simulink model "ES101A_DiagcMgr"  (R2013b)
settings: Solver=ode45  StartTime=0.0  StopTime=0.44  RelTol=1e-3
values from neighbouring files (symbols this model uses):
  BrdgVltg = DataDict.IpSignal    [ES101A_DiagcMgr_DataDict.m]
  DEM_CLEAR_PENDING = DataDict.Constant    [ES101A_DiagcMgr_DataDict.m]
  DEM_DTC_GROUP_ALL_DTCS = DataDict.Constant    [ES101A_DiagcMgr_DataDict.m]
  DFTAGICNTR_CNT_U08 = DataDict.Constant    [ES101A_DiagcMgr_DataDict.m]
  DIAGCMGR_NTCINFOSTSTESTFAILD_CNT_U08 = DataDict.Constant    [ES101A_DiagcMgrProxyX_DataDict.m]    (also in ES101A_DiagcMgr_DataDict.m)
  DIAGCMGR_NTCINFOSTSTESTFAILDTHISIGNCYC_CNT_U08 = DataDict.Constant    [ES101A_DiagcMgr_DataDict.m]
  DIAGCMGR_NTCINFOSTSTESTNOTCMPLTHISIGNCYC_CNT_U08 = DataDict.Constant    [ES101A_DiagcMgrProxyX_DataDict.m]    (also in ES101A_DiagcMgr_DataDict.m)
  DiagcMgrFltResp = DataDict.Calibration    [ES101A_DiagcMgrProxyX_DataDict.m]    (also in ES101A_DiagcMgr_DataDict.m)
  DiagcMgrNtcFltAry = DataDict.NVM    [ES101A_DiagcMgr_DataDict.m]
  DIAGCSTSCTRLDSHTDWNFLTPRSNT_CNT_U16 = DataDict.Constant    [ES101A_DiagcMgr_DataDict.m]
  DIAGCSTSDFTHWAG_CNT_U16 = DataDict.Constant    [ES101A_DiagcMgr_DataDict.m]
  DIAGCSTSDFTHWAGSERLCOMEXPRTVAL_CNT_U16 = DataDict.Constant    [ES101A_DiagcMgr_DataDict.m]
  DIAGCSTSDFTVEHSPD_CNT_U16 = DataDict.Constant    [ES101A_DiagcMgr_DataDict.m]
  DIAGCSTSININVAL_CNT_U16 = DataDict.Constant    [ES101A_DiagcMgrProxyX_DataDict.m]    (also in ES101A_DiagcMgr_DataDict.m)
  DIAGCSTSIVTR1INACTV_CNT_U16 = DataDict.Constant    [ES101A_DiagcMgr_DataDict.m]
  DIAGCSTSIVTR2INACTV_CNT_U16 = DataDict.Constant    [ES101A_DiagcMgr_DataDict.m]
  DIAGCSTSLIMDTPRFMNC_CNT_U16 = DataDict.Constant    [ES101A_DiagcMgr_DataDict.m]
  DIAGCSTSRAMPTOZEROFLTPRSNT_CNT_U16 = DataDict.Constant    [ES101A_DiagcMgr_DataDict.m]
  DIAGCSTSWHLIMBREJCTNDI_CNT_U16 = DataDict.Constant    [ES101A_DiagcMgr_DataDict.m]
  DTCIDXSTSFAIL_CNT_U08 = DataDict.Constant    [ES101A_DiagcMgr_DataDict.m]
  DTCIDXSTSNONTC_CNT_U08 = DataDict.Constant    [ES101A_DiagcMgr_DataDict.m]
  DTCIDXSTSNORES_CNT_U08 = DataDict.Constant    [ES101A_DiagcMgr_DataDict.m]
  DTCIDXSTSPASS_CNT_U08 = DataDict.Constant    [ES101A_DiagcMgr_DataDict.m]
  DTCIDXSTSUPDCFMD_CNT_U08 = DataDict.Constant    [ES101A_DiagcMgr_DataDict.m]
  ELECGLBPRM_IVTRCNT_CNT_U08 = DataDict.ConfigParam    [ES101A_DiagcMgrProxyX_DataDict.m]    (also in ES101A_DiagcMgr_DataDict.m)
  FLTINJ_DIAGCMGR_DIAGCSTSIVTR1INACTV = DataDict.Constant    [ES101A_DiagcMgr_DataDict.m]
  FLTINJ_DIAGCMGR_DIAGCSTSIVTR2INACTV = DataDict.Constant    [ES101A_DiagcMgr_DataDict.m]
  HwTq = DataDict.IpSignal    [ES101A_DiagcMgr_DataDict.m]
  IgnCntr = DataDict.IpSignal    [ES101A_DiagcMgr_DataDict.m]
  MAXDEBCNTRVAL_CNT_S16 = DataDict.Constant    [ES101A_DiagcMgr_DataDict.m]
  MAXRAMPRATE_ULSPERSEC_F32 = DataDict.Constant    [ES101A_DiagcMgrProxyX_DataDict.m]    (also in ES101A_DiagcMgr_DataDict.m)
  MINDEBCNTRVAL_CNT_S16 = DataDict.Constant    [ES101A_DiagcMgr_DataDict.m]
  MINRAMPRATE_ULSPERSEC_F32 = DataDict.Constant    [ES101A_DiagcMgrProxyX_DataDict.m]    (also in ES101A_DiagcMgr_DataDict.m)
  SCAMOTTQCMDTOONE_ULS_F32 = DataDict.Constant    [ES101A_DiagcMgrProxyX_DataDict.m]    (also in ES101A_DiagcMgr_DataDict.m)
  SCAMOTTQCMDTOZERO_ULS_F32 = DataDict.Constant    [ES101A_DiagcMgrProxyX_DataDict.m]    (also in ES101A_DiagcMgr_DataDict.m)
  SysSt = DataDict.IpSignal    [ES101A_DiagcMgr_DataDict.m]
  VehSpd = DataDict.IpSignal    [ES101A_DiagcMgr_DataDict.m]
undefined symbols (not defined in the file or in its folder): ActvMotTqCmdSca, ActvRampRate, AgiCntr, Dem_DTCFormatType, Dem_DTCOriginType, Dem_EventStatusType, DiagcData, DiagcMgrNtcMap, DiagcSts, DtcEnaMask, EcuT, HistNtcFltAry, MicroDiagcData, MotTq, NtcNr, NtcNrWithResd1, NtcStInfo, ProxySetNtcData, Sts, SysSt1, TOTNROFDTC_CNT_U08
libraries: simulink x149, FloatToFixd x5, NxtrNvM x3
(part 4 of 13)

== system ES101A_DiagcMgr/DiagcMgr/ReadNtcFltAry/Update DiagcMgrReadFltInfoAry and HistReadFltAry ==
  IC : Inport
  Add : Sum
  Bus Selector1 : BusSelector  OutputSignals=ApplIdx,NtcInfoIdx
  Compare To Constant : simulink/Logic and Bit Operations/Compare To Constant  relop=<  const=20  OutDataTypeStr=boolean
  Compare To Constant1 : simulink/Logic and Bit Operations/Compare To Constant  relop=<=  const=511  OutDataTypeStr=boolean
  Constant : Constant  OutDataTypeStr=uint8
  CopyRight2 : Subsystem  Description=|  mask(Copyright Information){none=on}
      | Copyright info block.                                               
      |                                                                     
      | Place copyright information at the top of every subsystem in design.
      mask prompts: none "No parameters"
      mask help: Place copyright information at the top of every subsystem in design.
      mask Display:
      | NxtrConf = 'Nexteer Confidential';
      | 
      | sys = bdroot; %handle for the current model ("system")
      | first = get_param(sys,'Created');
      | first = first(end-3:end);  %year is last four digits
      | 
      | last = get_param(sys,'LastModifiedDate');
      | if isempty(last)
      |     last = datestr(now,'yyyy');
      | else
      |     last = last(end-3:end);
      | end
      | 
      | if strcmp(first,last)
      |     fprintf('%s -- Copyright %s Nexteer',NxtrConf,first)
      | else
      |     fprintf('%s -- %s%s- %s Nexteer',NxtrConf,char(169),first,last)
      | end
  Data Store Read1 : DataStoreRead  DataStoreName=NtcMapIdx  DataStoreElements=NtcMapIdx
  Data Store Read2 : DataStoreRead  DataStoreName=DiagcMgrNtcMap  DataStoreElements=DiagcMgrNtcMap(:)
  Data Store Read3 : DataStoreRead  DataStoreName=ReadFltInfoIdx
  Data Store Read4 : DataStoreRead  DataStoreName=NtcMapIdx
  Data Store Write1 : DataStoreWrite  DataStoreName=NtcMapIdx
  For Number of NTCs : Subsystem  TreatAsAtomicUnit=on
  Logical Operator : Logic  AllPortsSameDT=off  OutDataTypeStr=boolean
  Selector1 : Selector  IndexMode=Zero-based  InputPortWidth=512  IndexOptions=Index vector (port)  Indices=[1 3]  OutputSizes=1
  While Iterator : WhileIterator  MaxIters=511  ShowIterationPort=on
  wires:
  Data Store Read2/1 -> Selector1/1
  Selector1/1 -> Bus Selector1/1
  While Iterator/1 -> For Number of NTCs/3(NtcMapIdx), Selector1/2
  Bus Selector1/1 -> For Number of NTCs/1(ApplIdx)  "<ApplIdx>"
  IC/1 -> While Iterator/2
  Logical Operator/1 -> While Iterator/1
  Add/1 -> Data Store Write1/1
  Constant/1 -> Add/2
  Data Store Read1/1 -> Add/1
  Data Store Read3/1 -> Compare To Constant/1
  Compare To Constant/1 -> Logical Operator/1
  Compare To Constant1/1 -> Logical Operator/2
  Data Store Read4/1 -> Compare To Constant1/1
  Bus Selector1/2 -> For Number of NTCs/2(NtcInfoIdx)  "<NtcInfoIdx>"

== system ES101A_DiagcMgr/DiagcMgr/ReadNtcFltAry/While((HistReadFltAryTempIdx < HistReadFltAryIdx) AND (ReadFltInfoIndx < 20)) ==
  IC : Inport
  Add1 : Sum  Inputs=+-
  Compare To Constant3 : simulink/Logic and Bit Operations/Compare To Constant  relop=<  const=0  OutDataTypeStr=boolean
  Compare To Constant5 : simulink/Logic and Bit Operations/Compare To Constant  relop=<=  const=20  OutDataTypeStr=boolean
  CopyRight1 : Subsystem  Description=|  mask(Copyright Information){none=on}
      | Copyright info block.                                               
      |                                                                     
      | Place copyright information at the top of every subsystem in design.
      mask prompts: none "No parameters"
      mask help: Place copyright information at the top of every subsystem in design.
      mask Display:
      | NxtrConf = 'Nexteer Confidential';
      | 
      | sys = bdroot; %handle for the current model ("system")
      | first = get_param(sys,'Created');
      | first = first(end-3:end);  %year is last four digits
      | 
      | last = get_param(sys,'LastModifiedDate');
      | if isempty(last)
      |     last = datestr(now,'yyyy');
      | else
      |     last = last(end-3:end);
      | end
      | 
      | if strcmp(first,last)
      |     fprintf('%s -- Copyright %s Nexteer',NxtrConf,first)
      | else
      |     fprintf('%s -- %s%s- %s Nexteer',NxtrConf,char(169),first,last)
      | end
  Data Store Read5 : DataStoreRead  DataStoreName=HistReadFltAryIdx
  Data Store Read7 : DataStoreRead  DataStoreName=ReadFltInfoIdx
  Data Store Read8 : DataStoreRead  DataStoreName=HistReadFltAryTempIdx
  Increment HistFltAryTempdx and NtcFltAryIdx : Subsystem  Priority=2
      settings: AttributesFormatString=Priority = %<Priority>
  Logical Operator1 : Logic  AllPortsSameDT=off  OutDataTypeStr=boolean
  Update NtcFltAry : Subsystem  Priority=1
      settings: AttributesFormatString=|
      | Priority = %<Priority>
      | %<Description>
  While Iterator : WhileIterator  MaxIters=20
  wires:
  IC/1 -> While Iterator/2
  Data Store Read8/1 -> Add1/1
  Data Store Read5/1 -> Add1/2
  Add1/1 -> Compare To Constant3/1
  Data Store Read7/1 -> Compare To Constant5/1
  Compare To Constant5/1 -> Logical Operator1/1
  Compare To Constant3/1 -> Logical Operator1/2
  Logical Operator1/1 -> While Iterator/1

== system ES101A_DiagcMgr/DiagcMgr/ReadNtcFltAry/While(ReadFltInfoIdx < TableSize[DiagcMgrReadFltInfoAry]) ==
  IC : Inport
  Compare To Constant2 : simulink/Logic and Bit Operations/Compare To Constant  relop=<  const=20  OutDataTypeStr=boolean
  CopyRight1 : Subsystem  Description=|  mask(Copyright Information){none=on}
      | Copyright info block.                                               
      |                                                                     
      | Place copyright information at the top of every subsystem in design.
      mask prompts: none "No parameters"
      mask help: Place copyright information at the top of every subsystem in design.
      mask Display:
      | NxtrConf = 'Nexteer Confidential';
      | 
      | sys = bdroot; %handle for the current model ("system")
      | first = get_param(sys,'Created');
      | first = first(end-3:end);  %year is last four digits
      | 
      | last = get_param(sys,'LastModifiedDate');
      | if isempty(last)
      |     last = datestr(now,'yyyy');
      | else
      |     last = last(end-3:end);
      | end
      | 
      | if strcmp(first,last)
      |     fprintf('%s -- Copyright %s Nexteer',NxtrConf,first)
      | else
      |     fprintf('%s -- %s%s- %s Nexteer',NxtrConf,char(169),first,last)
      | end
  Data Store Read6 : DataStoreRead  DataStoreName=ReadFltInfoIdx
  Increment Indices : Subsystem  Priority=2
      settings: AttributesFormatString=%<Priority>
  Update NtcFltAry : Subsystem  Priority=1
      settings: AttributesFormatString=%<Priority>
  While Iterator : WhileIterator  MaxIters=20
  wires:
  IC/1 -> While Iterator/2
  Data Store Read6/1 -> Compare To Constant2/1
  Compare To Constant2/1 -> While Iterator/1

== system ES101A_DiagcMgr/DiagcMgr/ReadNtcInfoAndDebCntr/ApplX ==
  note: This server runnable is designed such that any NTC of the type Non-Debounced
      | that is passed as an argument to this function will get a 0 value as its DebCntr.
      | DiagcMgr inherently does not store a unique DebCntr for Non-Debounced NTCs.
      | Hence the logic.
  NtcInfoIdx_ArgIn : Inport
  DebCntrIdx_ArgIn : Inport  Port=2
  Action Port : ActionPort  ActionType=case
  CopyRight2 : Subsystem  Description=|  mask(Copyright Information){none=on}
      | Copyright info block.                                               
      |                                                                     
      | Place copyright information at the top of every subsystem in design.
      mask prompts: none "No parameters"
      mask help: Place copyright information at the top of every subsystem in design.
      mask Display:
      | NxtrConf = 'Nexteer Confidential';
      | 
      | sys = bdroot; %handle for the current model ("system")
      | first = get_param(sys,'Created');
      | first = first(end-3:end);  %year is last four digits
      | 
      | last = get_param(sys,'LastModifiedDate');
      | if isempty(last)
      |     last = datestr(now,'yyyy');
      | else
      |     last = last(end-3:end);
      | end
      | 
      | if strcmp(first,last)
      |     fprintf('%s -- Copyright %s Nexteer',NxtrConf,first)
      | else
      |     fprintf('%s -- %s%s- %s Nexteer',NxtrConf,char(169),first,last)
      | end
  Debounced : Subsystem  TreatAsAtomicUnit=on
  GetNtcInfoAppIX : Subsystem  TreatAsAtomicUnit=on
  If1 : If  IfExpression=u1 == 0
  Merge : Merge
  NonDebounced : Subsystem  TreatAsAtomicUnit=on
  NtcInfo_ArgOut : Outport
  DebCntr_ArgOut : Outport  Port=2
  wires:
  NtcInfoIdx_ArgIn/1 -> GetNtcInfoAppIX/1(NtcInfoIdx_ArgIn)
  GetNtcInfoAppIX/1(NtcInfo_ArgOut) -> NtcInfo_ArgOut/1
  DebCntrIdx_ArgIn/1 -> If1/1, Debounced/1(DebCntrIdx_ArgIn)
  If1/1 -> NonDebounced/Action
  If1/2 -> Debounced/Action
  Merge/1 -> DebCntr_ArgOut/1
  NonDebounced/1(DebCntr_ArgOut) -> Merge/1
  Debounced/1(DebCntr_ArgOut) -> Merge/2

== system ES101A_DiagcMgr/DiagcMgr/ReadNtcInfoAndDebCntr/CopyRight2 ==

== system ES101A_DiagcMgr/DiagcMgr/ReadNtcInfoAndDebCntr/DoNothing ==
  Action Port : ActionPort
  CopyRight2 : Subsystem  Description=|  mask(Copyright Information){none=on}
      | Copyright info block.                                               
      |                                                                     
      | Place copyright information at the top of every subsystem in design.
      mask prompts: none "No parameters"
      mask help: Place copyright information at the top of every subsystem in design.
      mask Display:
      | NxtrConf = 'Nexteer Confidential';
      | 
      | sys = bdroot; %handle for the current model ("system")
      | first = get_param(sys,'Created');
      | first = first(end-3:end);  %year is last four digits
      | 
      | last = get_param(sys,'LastModifiedDate');
      | if isempty(last)
      |     last = datestr(now,'yyyy');
      | else
      |     last = last(end-3:end);
      | end
      | 
      | if strcmp(first,last)
      |     fprintf('%s -- Copyright %s Nexteer',NxtrConf,first)
      | else
      |     fprintf('%s -- %s%s- %s Nexteer',NxtrConf,char(169),first,last)
      | end

== system ES101A_DiagcMgr/DiagcMgr/ReadSnpshtData/CopyRight1 ==

== system ES101A_DiagcMgr/DiagcMgr/ReadSnpshtData/Send out data ==
  CopyRight2 : Subsystem  Description=|  mask(Copyright Information){none=on}
      | Copyright info block.                                               
      |                                                                     
      | Place copyright information at the top of every subsystem in design.
      mask prompts: none "No parameters"
      mask help: Place copyright information at the top of every subsystem in design.
      mask Display:
      | NxtrConf = 'Nexteer Confidential';
      | 
      | sys = bdroot; %handle for the current model ("system")
      | first = get_param(sys,'Created');
      | first = first(end-3:end);  %year is last four digits
      | 
      | last = get_param(sys,'LastModifiedDate');
      | if isempty(last)
      |     last = datestr(now,'yyyy');
      | else
      |     last = last(end-3:end);
      | end
      | 
      | if strcmp(first,last)
      |     fprintf('%s -- Copyright %s Nexteer',NxtrConf,first)
      | else
      |     fprintf('%s -- %s%s- %s Nexteer',NxtrConf,char(169),first,last)
      | end
  Data Store Read1 : DataStoreRead  DataStoreName=SnpshtDataAry
  ReadSnpshtAry_ArgOut : Outport
  wires:
  Data Store Read1/1 -> ReadSnpshtAry_ArgOut/1

== system ES101A_DiagcMgr/DiagcMgr/RestoreNtcFltAryDft/CopyRight2 ==

== system ES101A_DiagcMgr/DiagcMgr/RestoreNtcFltAryDft/Subsystem ==
  Length of NtcFltArray : Inport
  Assignment1 : Assignment  IndexMode=Zero-based  IndexOptions=Index vector (port)  Indices=1  OutputSizes=1
  Bus Assignment1 : BusAssignment  AssignedSignals=NtcNr,AgiCntr,Sts
  Constant1 : Constant  Value=0  OutDataTypeStr=uint16
  Constant2 : Constant  Value=DFTAGICNTR_CNT_U08  OutDataTypeStr=uint8
  Constant3 : Constant  Value=0  OutDataTypeStr=uint8
  CopyRight2 : Subsystem  Description=|  mask(Copyright Information){none=on}
      | Copyright info block.                                               
      |                                                                     
      | Place copyright information at the top of every subsystem in design.
      mask prompts: none "No parameters"
      mask help: Place copyright information at the top of every subsystem in design.
      mask Display:
      | NxtrConf = 'Nexteer Confidential';
      | 
      | sys = bdroot; %handle for the current model ("system")
      | first = get_param(sys,'Created');
      | first = first(end-3:end);  %year is last four digits
      | 
      | last = get_param(sys,'LastModifiedDate');
      | if isempty(last)
      |     last = datestr(now,'yyyy');
      | else
      |     last = last(end-3:end);
      | end
      | 
      | if strcmp(first,last)
      |     fprintf('%s -- Copyright %s Nexteer',NxtrConf,first)
      | else
      |     fprintf('%s -- %s%s- %s Nexteer',NxtrConf,char(169),first,last)
      | end
  Data Store Read1 : DataStoreRead  DataStoreName=DiagcMgrNtcFltAry  DataStoreElements=DiagcMgrNtcFltAry(:)
  Data Store Write2 : DataStoreWrite  DataStoreName=DiagcMgrNtcFltAry  DataStoreElements=DiagcMgrNtcFltAry(:)
  For Iterator : ForIterator  IterationSource=external  IndexMode=Zero-based
  Selector1 : Selector  IndexMode=Zero-based  InputPortWidth=20  IndexOptions=Index vector (port)  Indices=[1 3]  OutputSizes=1
  wires:
  Constant3/1 -> Bus Assignment1/4
  Constant2/1 -> Bus Assignment1/3
  Constant1/1 -> Bus Assignment1/2
  Length of NtcFltArray/1 -> For Iterator/1
  For Iterator/1 -> Selector1/2, Assignment1/3
  Bus Assignment1/1 -> Assignment1/2
  Assignment1/1 -> Data Store Write2/1
  Selector1/1 -> Bus Assignment1/1
  Data Store Read1/1 -> Selector1/1, Assignment1/1

== system ES101A_DiagcMgr/DiagcMgr/RestoreSnpshtAryDft/CopyRight2 ==

== system ES101A_DiagcMgr/DiagcMgr/RestoreSnpshtAryDft/Subsystem ==
  Length of Snapshot Array : Inport
  Assignment1 : Assignment  IndexMode=Zero-based  IndexOptions=Index vector (port)  Indices=1  OutputSizes=1
  Bus Assignment3 : BusAssignment  AssignedSignals=MicroDiagcData,HwTq,MotTq,IgnCntr,BrdgVltg,EcuT,NtcNr,NtcStInfo,SysSt,VehSpd
  Constant1 : Constant  Value=0  OutDataTypeStr=uint32
  Constant12 : Constant  Value=0  OutDataTypeStr=uint8
  Constant{2..4,7..8} (5 alike) : Constant  Value=0  OutDataTypeStr=single
  Constant5 : Constant  Value=SysSt1.SYSST_WRMININ  OutDataTypeStr=Enum: SysSt1
  Constant6 : Constant  Value=0  OutDataTypeStr=uint32
  Constant9 : Constant  Value=NtcNrWithResd1.NTCNR_RESD  OutDataTypeStr=Enum: NtcNrWithResd1
  CopyRight2 : Subsystem  Description=|  mask(Copyright Information){none=on}
      | Copyright info block.                                               
      |                                                                     
      | Place copyright information at the top of every subsystem in design.
      mask prompts: none "No parameters"
      mask help: Place copyright information at the top of every subsystem in design.
      mask Display:
      | NxtrConf = 'Nexteer Confidential';
      | 
      | sys = bdroot; %handle for the current model ("system")
      | first = get_param(sys,'Created');
      | first = first(end-3:end);  %year is last four digits
      | 
      | last = get_param(sys,'LastModifiedDate');
      | if isempty(last)
      |     last = datestr(now,'yyyy');
      | else
      |     last = last(end-3:end);
      | end
      | 
      | if strcmp(first,last)
      |     fprintf('%s -- Copyright %s Nexteer',NxtrConf,first)
      | else
      |     fprintf('%s -- %s%s- %s Nexteer',NxtrConf,char(169),first,last)
      | end
  Data Store Read1 : DataStoreRead  DataStoreName=SnpshtDataAry
  Data Store Write2 : DataStoreWrite  DataStoreName=SnpshtDataAry
  For Iterator : ForIterator  IterationSource=external  IndexMode=Zero-based  IterationVariableDataType=int16
  Selector1 : Selector  IndexMode=Zero-based  InputPortWidth=20  IndexOptions=Index vector (port)  Indices=[1 3]  OutputSizes=1
  wires:
  Data Store Read1/1 -> Assignment1/1, Selector1/1
  Selector1/1 -> Bus Assignment3/1
  Assignment1/1 -> Data Store Write2/1
  Bus Assignment3/1 -> Assignment1/2
  For Iterator/1 -> Assignment1/3, Selector1/2
  Length of Snapshot Array/1 -> For Iterator/1
  Constant1/1 -> Bus Assignment3/2
  Constant2/1 -> Bus Assignment3/3
  Constant9/1 -> Bus Assignment3/8
  Constant5/1 -> Bus Assignment3/10
  Constant12/1 -> Bus Assignment3/9
  Constant6/1 -> Bus Assignment3/5
  Constant7/1 -> Bus Assignment3/6
  Constant8/1 -> Bus Assignment3/7
  Constant3/1 -> Bus Assignment3/4
  Constant4/1 -> Bus Assignment3/11

== system ES101A_DiagcMgr/DiagcMgr/SetNtcStsCore/CopyRight2 ==

== system ES101A_DiagcMgr/DiagcMgr/SetNtcStsCore/Create SnapshotDataBus ==
  SysSt : Inport
  IgnCntr : Inport  Port=2
  RegInBRAMDAT1 : Inport  Port=3
  HwTq : Inport  Port=4
  MotTqCmdMrfScad : Inport  Port=5
  BrdgVltg : Inport  Port=6
  EcuTFild : Inport  Port=7
  VehSpd : Inport  Port=8
  Bus Creator : BusCreator  Inputs=8  OutDataTypeStr=Bus: SnpshtDataRec1
  CopyRight2 : Subsystem  Description=|  mask(Copyright Information){none=on}
      | Copyright info block.                                               
      |                                                                     
      | Place copyright information at the top of every subsystem in design.
      mask prompts: none "No parameters"
      mask help: Place copyright information at the top of every subsystem in design.
      mask Display:
      | NxtrConf = 'Nexteer Confidential';
      | 
      | sys = bdroot; %handle for the current model ("system")
      | first = get_param(sys,'Created');
      | first = first(end-3:end);  %year is last four digits
      | 
      | last = get_param(sys,'LastModifiedDate');
      | if isempty(last)
      |     last = datestr(now,'yyyy');
      | else
      |     last = last(end-3:end);
      | end
      | 
      | if strcmp(first,last)
      |     fprintf('%s -- Copyright %s Nexteer',NxtrConf,first)
      | else
      |     fprintf('%s -- %s%s- %s Nexteer',NxtrConf,char(169),first,last)
      | end
  FloatToFixd_s16_f1 : FloatToFixd/FloatToFixd_s16_f32  Param1=10
  FloatToFixd_s16_f3 : FloatToFixd/FloatToFixd_s16_f32  Param1=7
  FloatToFixd_s16_f32 : FloatToFixd/FloatToFixd_s16_f32  Param1=10
  FloatToFixd_u16_f1 : FloatToFixd/FloatToFixd_u16_f32  Param1=7
  FloatToFixd_u16_f32 : FloatToFixd/FloatToFixd_u16_f32  Param1=10
  SnapshotDataBus : Outport
  wires:
  SysSt/1 -> Bus Creator/7
  IgnCntr/1 -> Bus Creator/1
  RegInBRAMDAT1/1 -> Bus Creator/2
  HwTq/1 -> FloatToFixd_s16_f32/1
  MotTqCmdMrfScad/1 -> FloatToFixd_s16_f1/1
  BrdgVltg/1 -> FloatToFixd_u16_f32/1
  EcuTFild/1 -> FloatToFixd_s16_f3/1
  VehSpd/1 -> FloatToFixd_u16_f1/1
  Bus Creator/1 -> SnapshotDataBus/1
  FloatToFixd_s16_f32/1 -> Bus Creator/3
  FloatToFixd_s16_f1/1 -> Bus Creator/4
  FloatToFixd_u16_f32/1 -> Bus Creator/5
  FloatToFixd_s16_f3/1 -> Bus Creator/6
  FloatToFixd_u16_f1/1 -> Bus Creator/8

== system ES101A_DiagcMgr/DiagcMgr/SetNtcStsCore/NtcNr is Invalid ==
  Action Port : ActionPort  ActionType=else
  CopyRight2 : Subsystem  Description=|  mask(Copyright Information){none=on}
      | Copyright info block.                                               
      |                                                                     
      | Place copyright information at the top of every subsystem in design.
      mask prompts: none "No parameters"
      mask help: Place copyright information at the top of every subsystem in design.
      mask Display:
      | NxtrConf = 'Nexteer Confidential';
      | 
      | sys = bdroot; %handle for the current model ("system")
      | first = get_param(sys,'Created');
      | first = first(end-3:end);  %year is last four digits
      | 
      | last = get_param(sys,'LastModifiedDate');
      | if isempty(last)
      |     last = datestr(now,'yyyy');
      | else
      |     last = last(end-3:end);
      | end
      | 
      | if strcmp(first,last)
      |     fprintf('%s -- Copyright %s Nexteer',NxtrConf,first)
      | else
      |     fprintf('%s -- %s%s- %s Nexteer',NxtrConf,char(169),first,last)
      | end
  E_NOT_OK : Constant  OutDataTypeStr=uint8
  SetNtcSts_StdRtn : Outport
  wires:
  E_NOT_OK/1 -> SetNtcSts_StdRtn/1

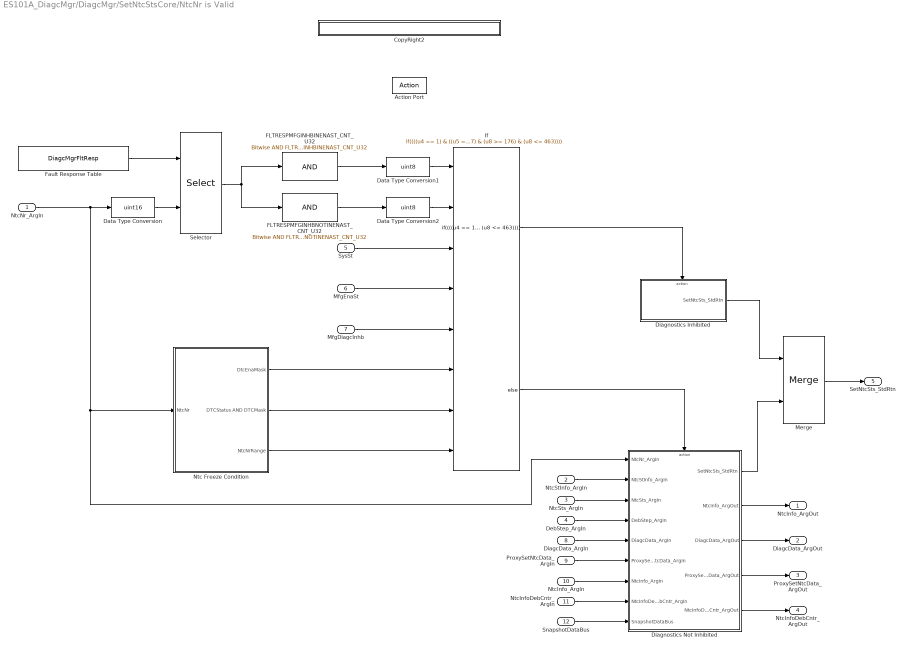
== system ES101A_DiagcMgr/DiagcMgr/SetNtcStsCore/NtcNr is Valid ==
  NtcNr_ArgIn : Inport  OutDataTypeStr=Enum: NtcNr1
  NtcStInfo_ArgIn : Inport  Port=2
  NtcSts_ArgIn : Inport  Port=3
  DebStep_ArgIn : Inport  Port=4
  SysSt : Inport  Port=5
  MfgEnaSt : Inport  Port=6
  MfgDiagcInhb : Inport  Port=7
  DiagcData_ArgIn : Inport  Port=8
  ProxySetNtcData_ArgIn : Inport  Port=9
  NtcInfo_ArgIn : Inport  Port=10
  NtcInfoDebCntr_ArgIn : Inport  Port=11
  SnapshotDataBus : Inport  Port=12
  Action Port : ActionPort  ActionType=then
  CopyRight2 : Subsystem  Description=|  mask(Copyright Information){none=on}
      | Copyright info block.                                               
      |                                                                     
      | Place copyright information at the top of every subsystem in design.
      mask prompts: none "No parameters"
      mask help: Place copyright information at the top of every subsystem in design.
      mask Display:
      | NxtrConf = 'Nexteer Confidential';
      | 
      | sys = bdroot; %handle for the current model ("system")
      | first = get_param(sys,'Created');
      | first = first(end-3:end);  %year is last four digits
      | 
      | last = get_param(sys,'LastModifiedDate');
      | if isempty(last)
      |     last = datestr(now,'yyyy');
      | else
      |     last = last(end-3:end);
      | end
      | 
      | if strcmp(first,last)
      |     fprintf('%s -- Copyright %s Nexteer',NxtrConf,first)
      | else
      |     fprintf('%s -- %s%s- %s Nexteer',NxtrConf,char(169),first,last)
      | end
  Data Type Conversion : DataTypeConversion  OutDataTypeStr=uint16
  Data Type Conversion1 : DataTypeConversion  OutDataTypeStr=uint8
  Data Type Conversion2 : DataTypeConversion  OutDataTypeStr=uint8
  Diagnostics Inhibited : Subsystem
  Diagnostics Not Inhibited : Subsystem  RequirementInfo="{'linktype_rmi_doors' '0000c474 (/ESG Group/FDD Module Requirements/EA4 Specific/ES101A_DiagcMgr)' '#ES101A_68' 'true' 'REQ:  ES101A_68' '' ; 'linktype_rmi_doors' '0000c474 (/ESG Group/FDD Module Requirements/EA4 Specific/ES101A_DiagcMgr)' '#ES101A_278' 'true' 'REQ:  ES101A_278' '' } %GIDa_b7a1320e_7113_43ee_9c12_2e59701a8c27"
  FLTRESPMFGINHBINENAST_CNT_U32 : simulink/Logic and Bit Operations/Bitwise Operator  RequirementInfo={} %GIDa_e3e71e30_edd6_46d9_83c6_38d60561c01e  logicop=AND  UseBitMask=on  BitMask=FLTRESPMFGINHBINENAST_CNT_U32  BitMaskRealWorld=Stored Integer
  FLTRESPMFGINHBNOTINENAST_CNT_U32 : simulink/Logic and Bit Operations/Bitwise Operator  RequirementInfo={} %GIDa_f5890cc9_815a_470c_bd58_76004367c247  logicop=AND  UseBitMask=on  BitMask=FLTRESPMFGINHBNOTINENAST_CNT_U32  BitMaskRealWorld=Stored Integer
  Fault Response Table : Constant  Value=DiagcMgrFltResp
  If : If  NumInputs=8  IfExpression=(((u4 == 1) & ((u5 == 1) & (u1 == 1)) | ((u2 == 1) & (u3 ~= 2))) | ((u6 ~= u7) & (u8 >= 176) & (u8 <= 463)))
  Merge : Merge
  Ntc Freeze Condition : Subsystem  RequirementInfo="{'linktype_rmi_doors' '0000c474 (/ESG Group/FDD Module Requirements/EA4 Specific/ES101A_DiagcMgr)' '#ES101A_306' 'true' 'REQ:  ES101A_306' '' ; 'linktype_rmi_doors' '0000c474 (/ESG Group/FDD Module Requirements/EA4 Specific/ES101A_DiagcMgr)' '#ES101A_316' 'true' 'REQ:  ES101A_316' '' } %GIDa_4961b6b2_f681_49a6_be60_c18be2f59728"
  Selector : Selector  IndexMode=Zero-based  InputPortWidth=512  IndexOptions=Index vector (port)  Indices=[1 3]  OutputSizes=1
  NtcInfo_ArgOut : Outport
  DiagcData_ArgOut : Outport  Port=2
  ProxySetNtcData_ArgOut : Outport  Port=3
  NtcInfoDebCntr_ArgOut : Outport  Port=4
  SetNtcSts_StdRtn : Outport  Port=5
  wires:
  NtcStInfo_ArgIn/1 -> Diagnostics Not Inhibited/2(NtcStInfo_ArgIn)
  NtcSts_ArgIn/1 -> Diagnostics Not Inhibited/3(NtcSts_ArgIn)
  DebStep_ArgIn/1 -> Diagnostics Not Inhibited/4(DebStep_ArgIn)
  Fault Response Table/1 -> Selector/1
  Selector/1 -> FLTRESPMFGINHBNOTINENAST_CNT_U32/1, FLTRESPMFGINHBINENAST_CNT_U32/1
  FLTRESPMFGINHBNOTINENAST_CNT_U32/1 -> Data Type Conversion2/1
  MfgEnaSt/1 -> If/4
  MfgDiagcInhb/1 -> If/5
  SysSt/1 -> If/3
  If/1 -> Diagnostics Inhibited/Action
  If/2 -> Diagnostics Not Inhibited/Action
  Data Type Conversion/1 -> Selector/2
  FLTRESPMFGINHBINENAST_CNT_U32/1 -> Data Type Conversion1/1
  Data Type Conversion1/1 -> If/1
  Data Type Conversion2/1 -> If/2
  DiagcData_ArgIn/1 -> Diagnostics Not Inhibited/5(DiagcData_ArgIn)
  ProxySetNtcData_ArgIn/1 -> Diagnostics Not Inhibited/6(ProxySetNtcData_ArgIn)
  NtcInfo_ArgIn/1 -> Diagnostics Not Inhibited/7(NtcInfo_ArgIn)
  Diagnostics Not Inhibited/2("NtcInfo_ArgOut ") -> NtcInfo_ArgOut/1
  Diagnostics Not Inhibited/3("DiagcData_ArgOut ") -> DiagcData_ArgOut/1
  Diagnostics Not Inhibited/4("ProxySetNtcData_ArgOut ") -> ProxySetNtcData_ArgOut/1
  NtcInfoDebCntr_ArgIn/1 -> Diagnostics Not Inhibited/8(NtcInfoDebCntr_ArgIn)
  Diagnostics Not Inhibited/5("NtcInfoDebCntr_ArgOut ") -> NtcInfoDebCntr_ArgOut/1
  Diagnostics Not Inhibited/1(SetNtcSts_StdRtn) -> Merge/2
  Diagnostics Inhibited/1(SetNtcSts_StdRtn) -> Merge/1
  Merge/1 -> SetNtcSts_StdRtn/1
  NtcNr_ArgIn/1 -> Diagnostics Not Inhibited/1(NtcNr_ArgIn), Ntc Freeze Condition/1(NtcNr), Data Type Conversion/1
  Ntc Freeze Condition/1(DtcEnaMask) -> If/6
  Ntc Freeze Condition/2(DTCStatus AND DTCMask) -> If/7
  Ntc Freeze Condition/3(NtcNrRange) -> If/8
  SnapshotDataBus/1 -> Diagnostics Not Inhibited/9(SnapshotDataBus)

== system ES101A_DiagcMgr/DiagcMgr/UpdDtcEnaCdn/ClrBit ==
  DtcEnaCdnId_ArgIn : Inport
  Action Port : ActionPort  ActionType=else
  Bitwise Operator : simulink/Logic and Bit Operations/Bitwise Operator  logicop=AND  UseBitMask=off  NumInputPorts=2  BitMask=bin2dec('11011001')  BitMaskRealWorld=Stored Integer
  Bitwise Operator1 : simulink/Logic and Bit Operations/Bitwise Operator  logicop=NOT  UseBitMask=off  BitMask=bin2dec('11011001')  BitMaskRealWorld=Stored Integer
  Constant : Constant  OutDataTypeStr=uint16
  CopyRight2 : Subsystem  Description=|  mask(Copyright Information){none=on}
      | Copyright info block.                                               
      |                                                                     
      | Place copyright information at the top of every subsystem in design.
      mask prompts: none "No parameters"
      mask help: Place copyright information at the top of every subsystem in design.
      mask Display:
      | NxtrConf = 'Nexteer Confidential';
      | 
      | sys = bdroot; %handle for the current model ("system")
      | first = get_param(sys,'Created');
      | first = first(end-3:end);  %year is last four digits
      | 
      | last = get_param(sys,'LastModifiedDate');
      | if isempty(last)
      |     last = datestr(now,'yyyy');
      | else
      |     last = last(end-3:end);
      | end
      | 
      | if strcmp(first,last)
      |     fprintf('%s -- Copyright %s Nexteer',NxtrConf,first)
      | else
      |     fprintf('%s -- %s%s- %s Nexteer',NxtrConf,char(169),first,last)
      | end
  Data Store Read : DataStoreRead  DataStoreName=DtcEnaSts
  Data Store Write : DataStoreWrite  DataStoreName=DtcEnaSts
  Shift Arithmetic : ArithShift  BitShiftNumberSource=Input port  BitShiftNumber=8  BitShiftDirection=Left
      settings: InputPortMap=u0,p1
  wires:
  DtcEnaCdnId_ArgIn/1 -> Shift Arithmetic/2
  Constant/1 -> Shift Arithmetic/1
  Bitwise Operator/1 -> Data Store Write/1
  Data Store Read/1 -> Bitwise Operator/1
  Shift Arithmetic/1 -> Bitwise Operator1/1
  Bitwise Operator1/1 -> Bitwise Operator/2

== system ES101A_DiagcMgr/DiagcMgr/UpdDtcEnaCdn/CopyRight2 ==

== system ES101A_DiagcMgr/DiagcMgr/UpdDtcEnaCdn/SetBit ==
  DtcEnaCdnId_ArgIn : Inport
  Action Port : ActionPort  ActionType=then
  Bitwise Operator : simulink/Logic and Bit Operations/Bitwise Operator  logicop=OR  UseBitMask=off  NumInputPorts=2  BitMask=bin2dec('11011001')  BitMaskRealWorld=Stored Integer
  Constant : Constant  OutDataTypeStr=uint16
  CopyRight2 : Subsystem  Description=|  mask(Copyright Information){none=on}
      | Copyright info block.                                               
      |                                                                     
      | Place copyright information at the top of every subsystem in design.
      mask prompts: none "No parameters"
      mask help: Place copyright information at the top of every subsystem in design.
      mask Display:
      | NxtrConf = 'Nexteer Confidential';
      | 
      | sys = bdroot; %handle for the current model ("system")
      | first = get_param(sys,'Created');
      | first = first(end-3:end);  %year is last four digits
      | 
      | last = get_param(sys,'LastModifiedDate');
      | if isempty(last)
      |     last = datestr(now,'yyyy');
      | else
      |     last = last(end-3:end);
      | end
      | 
      | if strcmp(first,last)
      |     fprintf('%s -- Copyright %s Nexteer',NxtrConf,first)
      | else
      |     fprintf('%s -- %s%s- %s Nexteer',NxtrConf,char(169),first,last)
      | end
  Data Store Read : DataStoreRead  DataStoreName=DtcEnaSts
  Data Store Write : DataStoreWrite  DataStoreName=DtcEnaSts
  Shift Arithmetic : ArithShift  BitShiftNumberSource=Input port  BitShiftNumber=8  BitShiftDirection=Left
      settings: InputPortMap=u0,p1
  wires:
  DtcEnaCdnId_ArgIn/1 -> Shift Arithmetic/2
  Constant/1 -> Shift Arithmetic/1
  Bitwise Operator/1 -> Data Store Write/1
  Data Store Read/1 -> Bitwise Operator/1
  Shift Arithmetic/1 -> Bitwise Operator/2

== system ES101A_DiagcMgr/DiagcMgr/ClrSnpshtData/Subsystem/CopyRight2 ==

== system ES101A_DiagcMgr/DiagcMgr/DiagcMgrIninCore/Initialize the NtcInfo Array/CopyRight2 ==

== system ES101A_DiagcMgr/DiagcMgr/DiagcMgrIninCore/Initialize the NtcInfo Array/Update the ISO bits of each NTC ==
  Number of Iteration : Inport
  NtcInfoAry_ArgIn : Inport  Port=2
  CopyRight2 : Subsystem  Description=|  mask(Copyright Information){none=on}
      | Copyright info block.                                               
      |                                                                     
      | Place copyright information at the top of every subsystem in design.
      mask prompts: none "No parameters"
      mask help: Place copyright information at the top of every subsystem in design.
      mask Display:
      | NxtrConf = 'Nexteer Confidential';
      | 
      | sys = bdroot; %handle for the current model ("system")
      | first = get_param(sys,'Created');
      | first = first(end-3:end);  %year is last four digits
      | 
      | last = get_param(sys,'LastModifiedDate');
      | if isempty(last)
      |     last = datestr(now,'yyyy');
      | else
      |     last = last(end-3:end);
      | end
      | 
      | if strcmp(first,last)
      |     fprintf('%s -- Copyright %s Nexteer',NxtrConf,first)
      | else
      |     fprintf('%s -- %s%s- %s Nexteer',NxtrConf,char(169),first,last)
      | end
  For Iterator : ForIterator  IterationSource=external  IterationLimit=22  IndexMode=Zero-based  IterationVariableDataType=int8
  Start Initialization : Subsystem  RequirementInfo="{'linktype_rmi_doors' '0000c474 (/ESG Group/FDD Module Requirements/EA4 Specific/ES101A_DiagcMgr)' '#ES101A_132' 'true' 'REQ:  ES101A_132' '' ; 'linktype_rmi_doors' '0000c474 (/ESG Group/FDD Module Requirements/EA4 Specific/ES101A_DiagcMgr)' '#ES101A_180' 'true' 'REQ:  ES101A_180' '' ; 'linktype_rmi_doors' '0000c474 (/ESG Group/FDD Module Requirements/EA4 Specific/ES101A_DiagcMgr)' '#ES101A_244' 'true' 'REQ:  ES101A_244' '' ; 'linktype_rmi_doors' '0000c474 (/ESG Group/FDD Module Requirements/EA4 Specific/ES101A_DiagcMgr)' '#ES101A_250' 'true' 'REQ:  ES101A_250' '' ; 'linktype_rmi_doors' '0000c474 (/ESG Group/FDD Module Requirements/EA4 Specific/ES101A_DiagcMgr)' '#ES101A_181' 'true' 'REQ:  ES101A_181' '' ; 'linktype_rmi_doors' '0000c474 (/ESG Group/FDD Module Requirements/EA4 Specific/ES101A_DiagcMgr)' '#ES101A_184' 'true' 'REQ:  ES101A_184' '' ; 'linktype_rmi_doors' '0000c474 (/ESG Group/FDD Module Requirements/EA4 Specific/ES101A_DiagcMgr)' '#ES101A_303' 'true' 'REQ:  ES101A_303' '' ; 'linktype_rmi_doors' '0000c474 (/ESG Group/FDD Module Requirements/EA4 Specific/ES101A_DiagcMgr)' '#ES101A_134' 'true' 'REQ:  ES101A_134' '' ; 'linktype_rmi_doors' '0000c474 (/ESG Group/FDD Module Requirements/EA4 Specific/ES101A_DiagcMgr)' '#ES101A_198' 'true' 'REQ:  ES101A_198' '' } %GIDa_7307835e_1e72_4461_aea7_7f9719f5946a"  TreatAsAtomicUnit=on
  NtcInfoAry_ArgOut : Outport
  wires:
  Number of Iteration/1 -> For Iterator/1
  For Iterator/1 -> Start Initialization/1(NtcInfoIdx)
  Start Initialization/1(NtcInfoAry_ArgOut) -> NtcInfoAry_ArgOut/1
  NtcInfoAry_ArgIn/1 -> Start Initialization/2(NtcInfoAry_ArgIn)

== system ES101A_DiagcMgr/DiagcMgr/DiagcMgrIninCore/Update DiagcSts and DiagcMgrActv/CopyRight2 ==

== system ES101A_DiagcMgr/DiagcMgr/DiagcMgrIninCore/Update DiagcSts and DiagcMgrActv/Dual Inverter ==
  Action Port : ActionPort  ActionType=else
  CopyRight2 : Subsystem  Description=|  mask(Copyright Information){none=on}
      | Copyright info block.                                               
      |                                                                     
      | Place copyright information at the top of every subsystem in design.
      mask prompts: none "No parameters"
      mask help: Place copyright information at the top of every subsystem in design.
      mask Display:
      | NxtrConf = 'Nexteer Confidential';
      | 
      | sys = bdroot; %handle for the current model ("system")
      | first = get_param(sys,'Created');
      | first = first(end-3:end);  %year is last four digits
      | 
      | last = get_param(sys,'LastModifiedDate');
      | if isempty(last)
      |     last = datestr(now,'yyyy');
      | else
      |     last = last(end-3:end);
      | end
      | 
      | if strcmp(first,last)
      |     fprintf('%s -- Copyright %s Nexteer',NxtrConf,first)
      | else
      |     fprintf('%s -- %s%s- %s Nexteer',NxtrConf,char(169),first,last)
      | end
  Inverter 2 Inactive : Constant  Value=DIAGCSTSININVAL_CNT_U16  OutDataTypeStr=uint16
  DiagcSts : Outport
  wires:
  Inverter 2 Inactive/1 -> DiagcSts/1

== system ES101A_DiagcMgr/DiagcMgr/DiagcMgrIninCore/Update DiagcSts and DiagcMgrActv/Single Inverter ==
  Action Port : ActionPort  ActionType=then
  CopyRight2 : Subsystem  Description=|  mask(Copyright Information){none=on}
      | Copyright info block.                                               
      |                                                                     
      | Place copyright information at the top of every subsystem in design.
      mask prompts: none "No parameters"
      mask help: Place copyright information at the top of every subsystem in design.
      mask Display:
      | NxtrConf = 'Nexteer Confidential';
      | 
      | sys = bdroot; %handle for the current model ("system")
      | first = get_param(sys,'Created');
      | first = first(end-3:end);  %year is last four digits
      | 
      | last = get_param(sys,'LastModifiedDate');
      | if isempty(last)
      |     last = datestr(now,'yyyy');
      | else
      |     last = last(end-3:end);
      | end
      | 
      | if strcmp(first,last)
      |     fprintf('%s -- Copyright %s Nexteer',NxtrConf,first)
      | else
      |     fprintf('%s -- %s%s- %s Nexteer',NxtrConf,char(169),first,last)
      | end
  Inverter 2 Inactive : Constant  Value=DIAGCSTSIVTR2INACTV_CNT_U16  OutDataTypeStr=uint16
  DiagcSts : Outport
  wires:
  Inverter 2 Inactive/1 -> DiagcSts/1

== system ES101A_DiagcMgr/DiagcMgr/DiagcMgrIninCore/Update NtcInfoAry From NvM/CopyRight2 ==

== system ES101A_DiagcMgr/DiagcMgr/DiagcMgrIninCore/Update NtcInfoAry From NvM/Update NtcInfoAry ==
  Length of NtcFltArray : Inport
  AppIdx_ArgIn : Inport  Port=2
  NtcInfoAry_ArgIn : Inport  Port=3
  CopyRight2 : Subsystem  Description=|  mask(Copyright Information){none=on}
      | Copyright info block.                                               
      |                                                                     
      | Place copyright information at the top of every subsystem in design.
      mask prompts: none "No parameters"
      mask help: Place copyright information at the top of every subsystem in design.
      mask Display:
      | NxtrConf = 'Nexteer Confidential';
      | 
      | sys = bdroot; %handle for the current model ("system")
      | first = get_param(sys,'Created');
      | first = first(end-3:end);  %year is last four digits
      | 
      | last = get_param(sys,'LastModifiedDate');
      | if isempty(last)
      |     last = datestr(now,'yyyy');
      | else
      |     last = last(end-3:end);
      | end
      | 
      | if strcmp(first,last)
      |     fprintf('%s -- Copyright %s Nexteer',NxtrConf,first)
      | else
      |     fprintf('%s -- %s%s- %s Nexteer',NxtrConf,char(169),first,last)
      | end
  For Iterator : ForIterator  IterationSource=external  IterationLimit=511  IndexMode=Zero-based  IterationVariableDataType=int8
  Update NtcInfoAry Aging Counter And Confirmed Bit : Subsystem  RequirementInfo={} %GIDa_5386584a_0950_4e1a_98bb_690191ebced3  TreatAsAtomicUnit=on
  NtcInfoAry_ArgOut : Outport
  wires:
  For Iterator/1 -> Update NtcInfoAry Aging Counter And Confirmed Bit/1(NtcFltIdx)
  Length of NtcFltArray/1 -> For Iterator/1
  AppIdx_ArgIn/1 -> Update NtcInfoAry Aging Counter And Confirmed Bit/2(AppIdx_ArgIn)
  NtcInfoAry_ArgIn/1 -> Update NtcInfoAry Aging Counter And Confirmed Bit/3(NtcInfoAry_ArgIn)
  Update NtcInfoAry Aging Counter And Confirmed Bit/1(NtcInfoAry_ArgOut) -> NtcInfoAry_ArgOut/1

== system ES101A_DiagcMgr/DiagcMgr/DiagcMgrPer1/Update OutpDiagcData/CopyRight2 ==

== system ES101A_DiagcMgr/DiagcMgr/DiagcMgrPer1/Update OutpDiagcData/GetDiagcDataApplX ==
  CopyRight2 : Subsystem  Description=|  mask(Copyright Information){none=on}
      | Copyright info block.                                               
      |                                                                     
      | Place copyright information at the top of every subsystem in design.
      mask prompts: none "No parameters"
      mask help: Place copyright information at the top of every subsystem in design.
      mask Display:
      | NxtrConf = 'Nexteer Confidential';
      | 
      | sys = bdroot; %handle for the current model ("system")
      | first = get_param(sys,'Created');
      | first = first(end-3:end);  %year is last four digits
      | 
      | last = get_param(sys,'LastModifiedDate');
      | if isempty(last)
      |     last = datestr(now,'yyyy');
      | else
      |     last = last(end-3:end);
      | end
      | 
      | if strcmp(first,last)
      |     fprintf('%s -- Copyright %s Nexteer',NxtrConf,first)
      | else
      |     fprintf('%s -- %s%s- %s Nexteer',NxtrConf,char(169),first,last)
      | end
  Ground : Ground
  TempDiagcData : Outport
  wires:
  Ground/1 -> TempDiagcData/1

== system ES101A_DiagcMgr/DiagcMgr/DiagcMgrPer1/Update the Reduced Performance Outputs/CopyRight2 ==

== system ES101A_DiagcMgr/DiagcMgr/DiagcMgrPer1/Update the Reduced Performance Outputs/FltInj_logl ==
  note: EA4.x Fault Injection
  note: This block requires no modification by FDD author.
      |
      | This block does not actually simulate any fault injection.  It is simply a pass-thru.
      |
      | Input port (#2) simply terminates its signal, but we are trying to force the FDD author
      | to properly use the FltInjectionLocType enumeration in FDD model.
  Sig : Inport
  "LocnKey  " : Inport  Port=2  OutDataTypeStr=uint16
  CopyRight1 : Subsystem  Description=|  mask(Copyright Information){none=on}
      | Copyright info block.                                               
      |                                                                     
      | Place copyright information at the top of every subsystem in design.
      mask prompts: none "No parameters"
      mask help: Place copyright information at the top of every subsystem in design.
      mask Display:
      | NxtrConf = 'Nexteer Confidential';
      | 
      | sys = bdroot; %handle for the current model ("system")
      | first = get_param(sys,'Created');
      | if(isempty(first))
      |     first = datestr(now,'yyyy');
      | else
      |     first = first(end-3:end);  %year is last four digits
      | end
      | 
      | last = get_param(sys,'LastModifiedDate');
      | if isempty(last)
      |     last = datestr(now,'yyyy');
      | else
      |     last = last(end-3:end);
      | end
      | 
      | if strcmp(first,last)
      |     fprintf('%s -- Copyright %s Nexteer',NxtrConf,first)
      | else
      |     fprintf('%s -- %s%s- %s Nexteer',NxtrConf,char(169),first,last)
      | end
  Terminator : Terminator
  Sig_Out : Outport
  wires:
  "LocnKey  "/1 -> Terminator/1
  Sig/1 -> Sig_Out/1

== system ES101A_DiagcMgr/DiagcMgr/DiagcMgrPer1/Update the Reduced Performance Outputs/FltInj_logl1 ==
  note: This block requires no modification by FDD author.
      |
      | This block does not actually simulate any fault injection.  It is simply a pass-thru.
      |
      | Input port (#2) simply terminates its signal, but we are trying to force the FDD author
      | to properly use the FltInjectionLocType enumeration in FDD model.
  note: EA4.x Fault Injection
  Sig : Inport
  "LocnKey  " : Inport  Port=2  OutDataTypeStr=uint16
  CopyRight1 : Subsystem  Description=|  mask(Copyright Information){none=on}
      | Copyright info block.                                               
      |                                                                     
      | Place copyright information at the top of every subsystem in design.
      mask prompts: none "No parameters"
      mask help: Place copyright information at the top of every subsystem in design.
      mask Display:
      | NxtrConf = 'Nexteer Confidential';
      | 
      | sys = bdroot; %handle for the current model ("system")
      | first = get_param(sys,'Created');
      | if(isempty(first))
      |     first = datestr(now,'yyyy');
      | else
      |     first = first(end-3:end);  %year is last four digits
      | end
      | 
      | last = get_param(sys,'LastModifiedDate');
      | if isempty(last)
      |     last = datestr(now,'yyyy');
      | else
      |     last = last(end-3:end);
      | end
      | 
      | if strcmp(first,last)
      |     fprintf('%s -- Copyright %s Nexteer',NxtrConf,first)
      | else
      |     fprintf('%s -- %s%s- %s Nexteer',NxtrConf,char(169),first,last)
      | end
  Terminator : Terminator
  Sig_Out : Outport
  wires:
  Sig/1 -> Sig_Out/1
  "LocnKey  "/1 -> Terminator/1

== system ES101A_DiagcMgr/DiagcMgr/DiagcMgrPer2/Clear All DTCs/Call DEM & Update DtcIdxPrevSts ==
  note: 1 - Primary
      | 2 - Mirror
      | 3 - Permanent
      | 4 - Secondary
      | Short term: DiagcMgr is currenlty planned to use the
      | Primary Memory. Might have to jump in again to clear the
      | different memories?
  note: 0 - OBD
      | 1 - UDS
      | 2 - J1939
      | Short term: DiagcMgr is currenlty planned to use the
      | UDS Format. Might have to jump in again to use the
      | different format?
  CopyRight2 : Subsystem  Description=|  mask(Copyright Information){none=on}
      | Copyright info block.                                               
      |                                                                     
      | Place copyright information at the top of every subsystem in design.
      mask prompts: none "No parameters"
      mask help: Place copyright information at the top of every subsystem in design.
      mask Display:
      | NxtrConf = 'Nexteer Confidential';
      | 
      | sys = bdroot; %handle for the current model ("system")
      | first = get_param(sys,'Created');
      | first = first(end-3:end);  %year is last four digits
      | 
      | last = get_param(sys,'LastModifiedDate');
      | if isempty(last)
      |     last = datestr(now,'yyyy');
      | else
      |     last = last(end-3:end);
      | end
      | 
      | if strcmp(first,last)
      |     fprintf('%s -- Copyright %s Nexteer',NxtrConf,first)
      | else
      |     fprintf('%s -- %s%s- %s Nexteer',NxtrConf,char(169),first,last)
      | end
  Dem_ClearDTC : Subsystem
  If : If  NumInputs=2  IfExpression=u1 ~= u2  ShowElse=off
  Primary Memory : Constant  Value=Dem_DTCOriginType.DEM_DTC_ORIGIN_PRIMARY_MEMORY
  Primary Memory1 : Constant  Value=DEM_DTC_GROUP_ALL_DTCS
  Primary Memory2 : Constant  Value=DEM_CLEAR_PENDING
  UDS : Constant  Value=Dem_DTCFormatType.DEM_DTC_FORMAT_UDS
  Update DtcIdxPrevSts and PrevClrDtcFlg : Subsystem  TreatAsAtomicUnit=on
  wires:
  UDS/1 -> Dem_ClearDTC/2(DTCFormat)
  Primary Memory/1 -> Dem_ClearDTC/3(DTCOrigin)
  Primary Memory1/1 -> Dem_ClearDTC/1(DTC)
  Dem_ClearDTC/1(Return) -> If/1
  Primary Memory2/1 -> If/2
  If/1 -> Update DtcIdxPrevSts and PrevClrDtcFlg/Action

== system ES101A_DiagcMgr/DiagcMgr/DiagcMgrPer2/Clear All DTCs/CopyRight2 ==

== system ES101A_DiagcMgr/DiagcMgr/DiagcMgrPer2/Normal Periodic Processing/CopyRight2 ==
